simulink model "corner_detection_2019b"  (R2024b)
settings: Solver=FixedStepDiscrete  StartTime=0.0  StopTime=0  RelTol=1e-3  EnableMultiTasking=on
undefined symbols (not defined in the file): fspecial, gray
libraries: visionanalysis x1, visiontextngfix x1, visionsources x1
settings Model: PacingRate=0.001800  Creator=FxMain  LastModifiedBy=AndreasK
settings SolverCC: AlgebraicLoopSolver=TrustRegion
settings DataIOCC: LimitDataPoints=on  SaveFormat=Array  ReturnWorkspaceOutputs=off
settings OptimizationCC: ExpressionDepthLimit=2147483647  LifeSpan=inf
settings DebuggingCC: UnderspecifiedInitializationDetection=Classic  MergeDetectMultiDrivingBlocksExec=none  SolverPrmCheckMsg=warning  FcnCallInpInsideContextMsg=warning  UnconnectedInputMsg=warning  UnconnectedOutputMsg=warning  UnconnectedLineMsg=warning  StateNameClashWarn=warning  SFUnexpectedBacktrackingDiag=warning  SFNoUnconditionalDefaultTransitionDiag=warning  SFExecutionAtInitializationDiag=none  ArithmeticOperatorsInVariantConditions=warning
settings HardwareCC: ProdBitPerPointer=32  ProdBitPerSizeT=32  ProdBitPerPtrDiffT=32  ProdLargestAtomicFloat=None  ProdIntDivRoundTo=Undefined  ProdEndianess=Unspecified  ProdWordSize=32  ProdHWDeviceType=32-bit Generic
settings ModelReferenceCC: EnableRefExpFcnMdlSchedulingChecks=on  PropagateSignalLabelsOutOfModel=off
settings SFSimCC: SimUseLocalCustomCode=off  CustomCodeUndefinedFunction=UseInterfaceOnly
settings RTWCC: RTWUseLocalCustomCode=off  GPUComputeCapability=3.5
settings CodeAppCC: StateflowObjectComments=on
settings GRTTargetCC: TargetLangStandard=C89/C90 (ANSI)  CombineOutputUpdateFcns=off  GRTInterface=on
settings ConfigComp: CovMetricSettings=dw  CovSaveCumulativeToWorkspaceVar=on  CovSaveSingleToWorkspaceVar=on  CovExternalEMLEnable=off

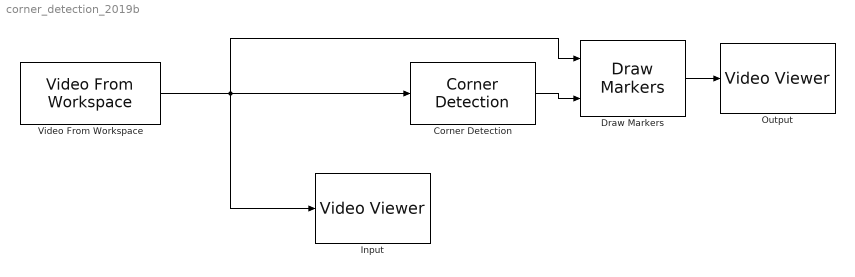
== system corner_detection_2019b ==
  Corner Detection : visionanalysis/Corner Detection  method=Minimum eigenvalue (Shi & Tomasi)  factor=0.04  filter=fspecial('gaussian', [1 5], 1.5)  thrInten=0.1  thrAngle=157.5  output=Obsolete9b  outputInUse=Corner location  maxNum=20  thrMetric=0.0005  neighborSize=[5 5]  isOutVarDim=on  roundingMode=Floor  overflowMode=off  firstCoeffMode=Specify word length  firstCoeffWordLength=16  firstCoeffFracLength=16  prodOutputMode=Binary point scaling  prodOutputWordLength=32  prodOutputFracLength=0  accumMode=Binary point scaling  accumWordLength=32  accumFracLength=0  memoryMode=Binary point scaling  memoryWordLength=32  memoryFracLength=0
  Draw Markers : visiontextngfix/Draw Markers  shape=Circle  size=20  fill=on  fillClrSource=Specify via dialog  display=White  intensity=200  color=255  opacity=0.6  viewport=Entire image  antialiasing=off  inType=Obsolete  imagePorts=One multidimensional signal  roundingMode=Floor  overflowMode=off  memoryMode=Specify word length  memoryWordLength=16  memoryFracLength=15  prodOutputMode=Binary point scaling  prodOutputWordLength=32  prodOutputFracLength=14
  Input : VideoViewer  colormapValue=gray(256)  FigPos=[272 748.4 992 635.4]
  Output : VideoViewer  colormapValue=gray(256)  FigPos=[211.4 776.4 1228 608]
  Video From Workspace : visionsources/Video From Workspace  signal=vid1  Ts=1  finalout=Obsolete  finaloutActive=Cyclic repetition  imagePorts=One multidimensional signal  OutPortLabels=R|G|B
  wires:
  Video From Workspace/1 -> Corner Detection/1, Input/1, Draw Markers/1
  Corner Detection/1 -> Draw Markers/2
  Draw Markers/1 -> Output/1
